simulink model "HybridFEMModel"  (Simulink 7.0)
settings: Solver=FixedStepDiscrete  SolverMode=SingleTasking  StartTime=0.0  StopTime=RunningTime  FixedStep=SampleRate  RelTol=1e-3
values from neighbouring files (symbols this model uses):
  SampleRate = Integrator.Timestep    [HybridFEMSetup_1.m]
undefined symbols (not defined in the file or in its folder): Elements
libraries: simulink x2
(part 2 of 2)

== matlab function Form Total Restoring Force Vector/Form Restoring Force Vector ==
  data: Nodes_muxed input inherited; RF_muxed input inherited; TotalRF output inherited
function TotalRF = eml(Nodes_muxed,RF_muxed)
% This block supports the Embedded MATLAB subset.
% See the help menu for details. 

NumFreeDOF = 12;
TotalRF = zeros(NumFreeDOF,1);

for i = 2:2:length(Nodes_muxed)
    N1 = Nodes_muxed(i-1);
    N2 = Nodes_muxed(i);
    if (3 * N1) <= NumFreeDOF
        TotalRF(N1 * 3 - 2, 1) = RF_muxed(1+(6*(i-2)/2)) + TotalRF(N1 * 3 - 2, 1);
        TotalRF(N1 * 3 - 1, 1) = RF_muxed(2+(6*(i-2)/2)) + TotalRF(N1 * 3 - 1, 1);
        TotalRF(N1 * 3, 1) = RF_muxed(3+(6*(i-2)/2)) + TotalRF(N1 * 3, 1);
    end
    if (3 * N2) <= NumFreeDOF
        TotalRF(N2 * 3 - 2, 1) = RF_muxed(4+(6*(i-2)/2)) + TotalRF(N2 * 3 - 2, 1);
        TotalRF(N2 * 3 - 1, 1) = RF_muxed(5+(6*(i-2)/2)) + TotalRF(N2 * 3 - 1, 1);
        TotalRF(N2 * 3, 1) = RF_muxed(6+(6*(i-2)/2)) + TotalRF(N2 * 3, 1);
    end
end

== matlab function Generate Type 1 Element Restoring Force/Type 1 Element RF ==
  data: Nodes output inherited; Element input inherited; RF output inherited; NumFreeDOF input inherited; Displacement input inherited
% get restoring force for the element
% returns (6x1) restoring force vector of element in global coordinates
function [Nodes,RF] = eml(Element, NumFreeDOF, Displacement)

%% Input mapping
Node1ID = Element(1);
Node1Xcoord = Element(2);
Node1Ycoord = Element(3);
Node2ID = Element(4);
Node2Xcoord = Element(5);
Node2Ycoord = Element(6);
MaterialE = Element(7);
Area = Element(8);
Inertia = Element(9);
Nodes = [Node1ID,Node2ID];

% Get distance between nodes
I1 = Node1ID;
I2 = Node2ID;
X21 = Node2Xcoord - Node1Xcoord;
Y21 = Node2Ycoord - Node1Ycoord;
EL = sqrt(X21 * X21 + Y21 * Y21);
EAL = MaterialE * Area / EL;
EIZL = MaterialE * Inertia / EL;
%calculation of density (the uniform load is only taken into account)
SEP = zeros(6);
SEP(1, 1) = EAL;
SEP(1, 4) = -EAL;
SEP(4, 4) = EAL;
SEP(2, 2) = 12 * EIZL / EL ^ 2;
SEP(2, 3) = 6 * EIZL / EL;
SEP(2, 5) = -SEP(2, 2);
SEP(2, 6) = SEP(2, 3);
SEP(3, 3) = 4 * EIZL;
SEP(3, 5) = -6 * EIZL / EL;
SEP(3, 6) = 2 * EIZL;
SEP(5, 5) = 12 * EIZL / EL ^ 2;
SEP(5, 6) = -6 * EIZL / EL;
SEP(6, 6) = 4 * EIZL;
for i = 1:6
   for j = i:6
      SEP(j, i) = SEP(i, j);
   end
end
DCOS = zeros(3,3);
DCOS(1, 1) = X21 / EL;
DCOS(1, 2) = Y21 / EL;
DCOS(1, 3) = 0;
DCOS(2, 1) = -DCOS(1, 2);
DCOS(2, 2) = DCOS(1, 1);
DCOS(2, 3) = 0;
DCOS(3, 1) = 0;
DCOS(3, 2) = 0;
DCOS(3, 3) = 1;
ALMBDA = zeros(6);       
for i = 1:2
   IK = 3 * (i - 1);
   for j = 1:3
      for k = 1:3
         ALMBDA(j + IK, k + IK) = DCOS(j, k);
      end
   end
end
SE = SEP * ALMBDA;
SEP = SE;
SE = ALMBDA' * SEP;
%create the displacement Ue (6x1) vector of the element in global coordinates
Ue = zeros(6,1);
if (I1 * 3) <= NumFreeDOF
    Ue(1, 1) = Displacement(I1 * 3 - 2, 1);
    Ue(2, 1) = Displacement(I1 * 3 - 1, 1);
    Ue(3, 1) = Displacement(I1 * 3, 1);
end
if (I2 * 3) <= NumFreeDOF
    Ue(4, 1) = Displacement(I2 * 3 - 2, 1);
    Ue(5, 1) = Displacement(I2 * 3 - 1, 1);
    Ue(6, 1) = Displacement(I2 * 3, 1);
end
RF = SE * Ue;  %resisting (6x1) resisting force vector of element in global coordinates

== matlab function Generate Type 1 Element Restoring Force1/Type 1 Element RF ==
  data: Nodes output inherited; Element input inherited; RF output inherited; NumFreeDOF input inherited; Displacement input inherited
% get restoring force for the element
% returns (6x1) restoring force vector of element in global coordinates
function [Nodes,RF] = eml(Element, NumFreeDOF, Displacement)

%% Input mapping
Node1ID = Element(1);
Node1Xcoord = Element(2);
Node1Ycoord = Element(3);
Node2ID = Element(4);
Node2Xcoord = Element(5);
Node2Ycoord = Element(6);
MaterialE = Element(7);
Area = Element(8);
Inertia = Element(9);
Nodes = [Node1ID,Node2ID];

% Get distance between nodes
I1 = Node1ID;
I2 = Node2ID;
X21 = Node2Xcoord - Node1Xcoord;
Y21 = Node2Ycoord - Node1Ycoord;
EL = sqrt(X21 * X21 + Y21 * Y21);
EAL = MaterialE * Area / EL;
EIZL = MaterialE * Inertia / EL;
%calculation of density (the uniform load is only taken into account)
SEP = zeros(6);
SEP(1, 1) = EAL;
SEP(1, 4) = -EAL;
SEP(4, 4) = EAL;
SEP(2, 2) = 12 * EIZL / EL ^ 2;
SEP(2, 3) = 6 * EIZL / EL;
SEP(2, 5) = -SEP(2, 2);
SEP(2, 6) = SEP(2, 3);
SEP(3, 3) = 4 * EIZL;
SEP(3, 5) = -6 * EIZL / EL;
SEP(3, 6) = 2 * EIZL;
SEP(5, 5) = 12 * EIZL / EL ^ 2;
SEP(5, 6) = -6 * EIZL / EL;
SEP(6, 6) = 4 * EIZL;
for i = 1:6
   for j = i:6
      SEP(j, i) = SEP(i, j);
   end
end
DCOS = zeros(3,3);
DCOS(1, 1) = X21 / EL;
DCOS(1, 2) = Y21 / EL;
DCOS(1, 3) = 0;
DCOS(2, 1) = -DCOS(1, 2);
DCOS(2, 2) = DCOS(1, 1);
DCOS(2, 3) = 0;
DCOS(3, 1) = 0;
DCOS(3, 2) = 0;
DCOS(3, 3) = 1;
ALMBDA = zeros(6);       
for i = 1:2
   IK = 3 * (i - 1);
   for j = 1:3
      for k = 1:3
         ALMBDA(j + IK, k + IK) = DCOS(j, k);
      end
   end
end
SE = SEP * ALMBDA;
SEP = SE;
SE = ALMBDA' * SEP;
%create the displacement Ue (6x1) vector of the element in global coordinates
Ue = zeros(6,1);
if (I1 * 3) <= NumFreeDOF
    Ue(1, 1) = Displacement(I1 * 3 - 2, 1);
    Ue(2, 1) = Displacement(I1 * 3 - 1, 1);
    Ue(3, 1) = Displacement(I1 * 3, 1);
end
if (I2 * 3) <= NumFreeDOF
    Ue(4, 1) = Displacement(I2 * 3 - 2, 1);
    Ue(5, 1) = Displacement(I2 * 3 - 1, 1);
    Ue(6, 1) = Displacement(I2 * 3, 1);
end
RF = SE * Ue;  %resisting (6x1) resisting force vector of element in global coordinates

== matlab function Generate Type 1 Element Restoring Force2/Type 1 Element RF ==
  data: Nodes output inherited; Element input inherited; RF output inherited; NumFreeDOF input inherited; Displacement input inherited
% get restoring force for the element
% returns (6x1) restoring force vector of element in global coordinates
function [Nodes,RF] = eml(Element, NumFreeDOF, Displacement)

%% Input mapping
Node1ID = Element(1);
Node1Xcoord = Element(2);
Node1Ycoord = Element(3);
Node2ID = Element(4);
Node2Xcoord = Element(5);
Node2Ycoord = Element(6);
MaterialE = Element(7);
Area = Element(8);
Inertia = Element(9);
Nodes = [Node1ID,Node2ID];

% Get distance between nodes
I1 = Node1ID;
I2 = Node2ID;
X21 = Node2Xcoord - Node1Xcoord;
Y21 = Node2Ycoord - Node1Ycoord;
EL = sqrt(X21 * X21 + Y21 * Y21);
EAL = MaterialE * Area / EL;
EIZL = MaterialE * Inertia / EL;
%calculation of density (the uniform load is only taken into account)
SEP = zeros(6);
SEP(1, 1) = EAL;
SEP(1, 4) = -EAL;
SEP(4, 4) = EAL;
SEP(2, 2) = 12 * EIZL / EL ^ 2;
SEP(2, 3) = 6 * EIZL / EL;
SEP(2, 5) = -SEP(2, 2);
SEP(2, 6) = SEP(2, 3);
SEP(3, 3) = 4 * EIZL;
SEP(3, 5) = -6 * EIZL / EL;
SEP(3, 6) = 2 * EIZL;
SEP(5, 5) = 12 * EIZL / EL ^ 2;
SEP(5, 6) = -6 * EIZL / EL;
SEP(6, 6) = 4 * EIZL;
for i = 1:6
   for j = i:6
      SEP(j, i) = SEP(i, j);
   end
end
DCOS = zeros(3,3);
DCOS(1, 1) = X21 / EL;
DCOS(1, 2) = Y21 / EL;
DCOS(1, 3) = 0;
DCOS(2, 1) = -DCOS(1, 2);
DCOS(2, 2) = DCOS(1, 1);
DCOS(2, 3) = 0;
DCOS(3, 1) = 0;
DCOS(3, 2) = 0;
DCOS(3, 3) = 1;
ALMBDA = zeros(6);       
for i = 1:2
   IK = 3 * (i - 1);
   for j = 1:3
      for k = 1:3
         ALMBDA(j + IK, k + IK) = DCOS(j, k);
      end
   end
end
SE = SEP * ALMBDA;
SEP = SE;
SE = ALMBDA' * SEP;
%create the displacement Ue (6x1) vector of the element in global coordinates
Ue = zeros(6,1);
if (I1 * 3) <= NumFreeDOF
    Ue(1, 1) = Displacement(I1 * 3 - 2, 1);
    Ue(2, 1) = Displacement(I1 * 3 - 1, 1);
    Ue(3, 1) = Displacement(I1 * 3, 1);
end
if (I2 * 3) <= NumFreeDOF
    Ue(4, 1) = Displacement(I2 * 3 - 2, 1);
    Ue(5, 1) = Displacement(I2 * 3 - 1, 1);
    Ue(6, 1) = Displacement(I2 * 3, 1);
end
RF = SE * Ue;  %resisting (6x1) resisting force vector of element in global coordinates

== matlab function Generate Type 1 Element Restoring Force3/Type 1 Element RF ==
  data: Nodes output inherited; Element input inherited; RF output inherited; NumFreeDOF input inherited; Displacement input inherited
% get restoring force for the element
% returns (6x1) restoring force vector of element in global coordinates
function [Nodes,RF] = eml(Element, NumFreeDOF, Displacement)

%% Input mapping
Node1ID = Element(1);
Node1Xcoord = Element(2);
Node1Ycoord = Element(3);
Node2ID = Element(4);
Node2Xcoord = Element(5);
Node2Ycoord = Element(6);
MaterialE = Element(7);
Area = Element(8);
Inertia = Element(9);
Nodes = [Node1ID,Node2ID];

% Get distance between nodes
I1 = Node1ID;
I2 = Node2ID;
X21 = Node2Xcoord - Node1Xcoord;
Y21 = Node2Ycoord - Node1Ycoord;
EL = sqrt(X21 * X21 + Y21 * Y21);
EAL = MaterialE * Area / EL;
EIZL = MaterialE * Inertia / EL;
%calculation of density (the uniform load is only taken into account)
SEP = zeros(6);
SEP(1, 1) = EAL;
SEP(1, 4) = -EAL;
SEP(4, 4) = EAL;
SEP(2, 2) = 12 * EIZL / EL ^ 2;
SEP(2, 3) = 6 * EIZL / EL;
SEP(2, 5) = -SEP(2, 2);
SEP(2, 6) = SEP(2, 3);
SEP(3, 3) = 4 * EIZL;
SEP(3, 5) = -6 * EIZL / EL;
SEP(3, 6) = 2 * EIZL;
SEP(5, 5) = 12 * EIZL / EL ^ 2;
SEP(5, 6) = -6 * EIZL / EL;
SEP(6, 6) = 4 * EIZL;
for i = 1:6
   for j = i:6
      SEP(j, i) = SEP(i, j);
   end
end
DCOS = zeros(3,3);
DCOS(1, 1) = X21 / EL;
DCOS(1, 2) = Y21 / EL;
DCOS(1, 3) = 0;
DCOS(2, 1) = -DCOS(1, 2);
DCOS(2, 2) = DCOS(1, 1);
DCOS(2, 3) = 0;
DCOS(3, 1) = 0;
DCOS(3, 2) = 0;
DCOS(3, 3) = 1;
ALMBDA = zeros(6);       
for i = 1:2
   IK = 3 * (i - 1);
   for j = 1:3
      for k = 1:3
         ALMBDA(j + IK, k + IK) = DCOS(j, k);
      end
   end
end
SE = SEP * ALMBDA;
SEP = SE;
SE = ALMBDA' * SEP;
%create the displacement Ue (6x1) vector of the element in global coordinates
Ue = zeros(6,1);
if (I1 * 3) <= NumFreeDOF
    Ue(1, 1) = Displacement(I1 * 3 - 2, 1);
    Ue(2, 1) = Displacement(I1 * 3 - 1, 1);
    Ue(3, 1) = Displacement(I1 * 3, 1);
end
if (I2 * 3) <= NumFreeDOF
    Ue(4, 1) = Displacement(I2 * 3 - 2, 1);
    Ue(5, 1) = Displacement(I2 * 3 - 1, 1);
    Ue(6, 1) = Displacement(I2 * 3, 1);
end
RF = SE * Ue;  %resisting (6x1) resisting force vector of element in global coordinates

== matlab function Generate Type 1 Element Restoring Force4/Type 1 Element RF ==
  data: Nodes output inherited; Element input inherited; RF output inherited; NumFreeDOF input inherited; Displacement input inherited
% get restoring force for the element
% returns (6x1) restoring force vector of element in global coordinates
function [Nodes,RF] = eml(Element, NumFreeDOF, Displacement)

%% Input mapping
Node1ID = Element(1);
Node1Xcoord = Element(2);
Node1Ycoord = Element(3);
Node2ID = Element(4);
Node2Xcoord = Element(5);
Node2Ycoord = Element(6);
MaterialE = Element(7);
Area = Element(8);
Inertia = Element(9);
Nodes = [Node1ID,Node2ID];

% Get distance between nodes
I1 = Node1ID;
I2 = Node2ID;
X21 = Node2Xcoord - Node1Xcoord;
Y21 = Node2Ycoord - Node1Ycoord;
EL = sqrt(X21 * X21 + Y21 * Y21);
EAL = MaterialE * Area / EL;
EIZL = MaterialE * Inertia / EL;
%calculation of density (the uniform load is only taken into account)
SEP = zeros(6);
SEP(1, 1) = EAL;
SEP(1, 4) = -EAL;
SEP(4, 4) = EAL;
SEP(2, 2) = 12 * EIZL / EL ^ 2;
SEP(2, 3) = 6 * EIZL / EL;
SEP(2, 5) = -SEP(2, 2);
SEP(2, 6) = SEP(2, 3);
SEP(3, 3) = 4 * EIZL;
SEP(3, 5) = -6 * EIZL / EL;
SEP(3, 6) = 2 * EIZL;
SEP(5, 5) = 12 * EIZL / EL ^ 2;
SEP(5, 6) = -6 * EIZL / EL;
SEP(6, 6) = 4 * EIZL;
for i = 1:6
   for j = i:6
      SEP(j, i) = SEP(i, j);
   end
end
DCOS = zeros(3,3);
DCOS(1, 1) = X21 / EL;
DCOS(1, 2) = Y21 / EL;
DCOS(1, 3) = 0;
DCOS(2, 1) = -DCOS(1, 2);
DCOS(2, 2) = DCOS(1, 1);
DCOS(2, 3) = 0;
DCOS(3, 1) = 0;
DCOS(3, 2) = 0;
DCOS(3, 3) = 1;
ALMBDA = zeros(6);       
for i = 1:2
   IK = 3 * (i - 1);
   for j = 1:3
      for k = 1:3
         ALMBDA(j + IK, k + IK) = DCOS(j, k);
      end
   end
end
SE = SEP * ALMBDA;
SEP = SE;
SE = ALMBDA' * SEP;
%create the displacement Ue (6x1) vector of the element in global coordinates
Ue = zeros(6,1);
if (I1 * 3) <= NumFreeDOF
    Ue(1, 1) = Displacement(I1 * 3 - 2, 1);
    Ue(2, 1) = Displacement(I1 * 3 - 1, 1);
    Ue(3, 1) = Displacement(I1 * 3, 1);
end
if (I2 * 3) <= NumFreeDOF
    Ue(4, 1) = Displacement(I2 * 3 - 2, 1);
    Ue(5, 1) = Displacement(I2 * 3 - 1, 1);
    Ue(6, 1) = Displacement(I2 * 3, 1);
end
RF = SE * Ue;  %resisting (6x1) resisting force vector of element in global coordinates

== matlab function Generate Type 1 Element Restoring Force5/Type 1 Element RF ==
  data: Nodes output inherited; Element input inherited; RF output inherited; NumFreeDOF input inherited; Displacement input inherited
% get restoring force for the element
% returns (6x1) restoring force vector of element in global coordinates
function [Nodes,RF] = eml(Element, NumFreeDOF, Displacement)

%% Input mapping
Node1ID = Element(1);
Node1Xcoord = Element(2);
Node1Ycoord = Element(3);
Node2ID = Element(4);
Node2Xcoord = Element(5);
Node2Ycoord = Element(6);
MaterialE = Element(7);
Area = Element(8);
Inertia = Element(9);
Nodes = [Node1ID,Node2ID];

% Get distance between nodes
I1 = Node1ID;
I2 = Node2ID;
X21 = Node2Xcoord - Node1Xcoord;
Y21 = Node2Ycoord - Node1Ycoord;
EL = sqrt(X21 * X21 + Y21 * Y21);
EAL = MaterialE * Area / EL;
EIZL = MaterialE * Inertia / EL;
%calculation of density (the uniform load is only taken into account)
SEP = zeros(6);
SEP(1, 1) = EAL;
SEP(1, 4) = -EAL;
SEP(4, 4) = EAL;
SEP(2, 2) = 12 * EIZL / EL ^ 2;
SEP(2, 3) = 6 * EIZL / EL;
SEP(2, 5) = -SEP(2, 2);
SEP(2, 6) = SEP(2, 3);
SEP(3, 3) = 4 * EIZL;
SEP(3, 5) = -6 * EIZL / EL;
SEP(3, 6) = 2 * EIZL;
SEP(5, 5) = 12 * EIZL / EL ^ 2;
SEP(5, 6) = -6 * EIZL / EL;
SEP(6, 6) = 4 * EIZL;
for i = 1:6
   for j = i:6
      SEP(j, i) = SEP(i, j);
   end
end
DCOS = zeros(3,3);
DCOS(1, 1) = X21 / EL;
DCOS(1, 2) = Y21 / EL;
DCOS(1, 3) = 0;
DCOS(2, 1) = -DCOS(1, 2);
DCOS(2, 2) = DCOS(1, 1);
DCOS(2, 3) = 0;
DCOS(3, 1) = 0;
DCOS(3, 2) = 0;
DCOS(3, 3) = 1;
ALMBDA = zeros(6);       
for i = 1:2
   IK = 3 * (i - 1);
   for j = 1:3
      for k = 1:3
         ALMBDA(j + IK, k + IK) = DCOS(j, k);
      end
   end
end
SE = SEP * ALMBDA;
SEP = SE;
SE = ALMBDA' * SEP;
%create the displacement Ue (6x1) vector of the element in global coordinates
Ue = zeros(6,1);
if (I1 * 3) <= NumFreeDOF
    Ue(1, 1) = Displacement(I1 * 3 - 2, 1);
    Ue(2, 1) = Displacement(I1 * 3 - 1, 1);
    Ue(3, 1) = Displacement(I1 * 3, 1);
end
if (I2 * 3) <= NumFreeDOF
    Ue(4, 1) = Displacement(I2 * 3 - 2, 1);
    Ue(5, 1) = Displacement(I2 * 3 - 1, 1);
    Ue(6, 1) = Displacement(I2 * 3, 1);
end
RF = SE * Ue;  %resisting (6x1) resisting force vector of element in global coordinates

== matlab function Generate Acceleration Vector/Generate Acceleration Vector ==
  data: TotalRF input inherited; PEFF input inherited; M_FreeInv input inherited; Acceleration output inherited; C_Free input inherited; Velocity input inherited; step_count input inherited
function Acceleration = eml(TotalRF,PEFF,M_FreeInv,C_Free,Velocity,step_count)
% This block supports the Embedded MATLAB subset.
% See the help menu for details. 

Acceleration = M_FreeInv * (PEFF(step_count,:)' - C_Free * Velocity - TotalRF);

== matlab function Generate Command Vectors/Generate Command Vectors ==
  data: Timestep input inherited; Displacement_v output inherited; Beta1 input inherited; Beta2 input inherited; Displacement input inherited; Velocity input inherited; Acceleration input inherited; Velocity_v output inherited
function [Displacement_v,Velocity_v] = eml(Timestep, Beta1, Beta2, Displacement, Velocity, Acceleration)
% This block supports the Embedded MATLAB subset.
% See the help menu for details. 

Displacement_v = Displacement + Timestep*Velocity + Beta2*Timestep^2*Acceleration;
Velocity_v = Velocity + Beta1*Timestep*Acceleration;
